simulink model "Fig32"  (R2014b)
settings: Solver=ode3  StartTime=0.0  StopTime=.005  FixedStep=2e-5  RelTol=1e-3
undefined symbols (not defined in the file or in its folder): tau
libraries: commfilt2 x2
settings Model: Creator=Dennis Silage  LastModifiedBy=Silage
settings DataIOCC: SignalLoggingSaveFormat=ModelDataLogs
settings OptimizationCC: ExpressionDepthLimit=2147483647  InitFltsAndDblsToZero=on
settings DebuggingCC: UnderspecifiedInitializationDetection=Classic  MergeDetectMultiDrivingBlocksExec=none  FcnCallInpInsideContextMsg=UseLocalSettings  StateNameClashWarn=warning  StrictBusMsg=Warning
settings GRTTargetCC: CombineOutputUpdateFcns=off  GRTInterface=on

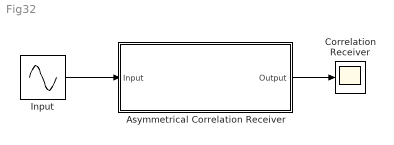
== system Fig32 ==
  "Asymmetrical Correlation Receiver " : Subsystem
  Correlation Receiver : Scope
      settings: YMin=0  YMax=30
  Input : Sin  Frequency=3141.5926  SampleTime=20e-6
  wires:
  Input/1 -> "Asymmetrical Correlation Receiver "/1(Input)
  "Asymmetrical Correlation Receiver "/1(Output) -> Correlation Receiver/1

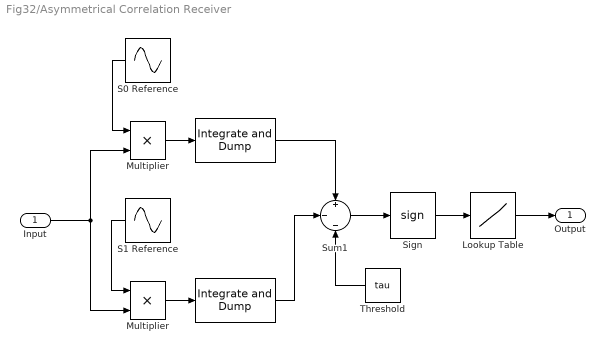
== system Fig32/Asymmetrical Correlation Receiver  ==
  Input : Inport
  " " : commfilt2/Integrate and Dump  obssamples=50  offsetsamples=0  nodump=off  roundingMode=Floor  overflowMode=off
  "   " : commfilt2/Integrate and Dump  obssamples=50  offsetsamples=0  nodump=off  roundingMode=Floor  overflowMode=off
  Lookup Table : Lookup  InputValues=[-1,0,1]  Table=[-1,-1,1]
  Multiplier : Product  RndMeth=Zero
  "Multiplier " : Product  RndMeth=Zero
  S0 Reference : Sin  Frequency=3141.59  SampleTime=20e-6  VectorParams1D=off
  S1 Reference : Sin  Frequency=3141.59  SampleTime=20e-6  VectorParams1D=off
  Sign : Signum
  Sum1 : Sum  Inputs=+|-|-
  Threshold : Constant  Value=tau
  Output : Outport
  wires:
  Multiplier/1 -> " "/1
  S0 Reference/1 -> Multiplier/1
  Input/1 -> Multiplier/2, "Multiplier "/2
  Sign/1 -> Lookup Table/1
  "Multiplier "/1 -> "   "/1
  Sum1/1 -> Sign/1
  Lookup Table/1 -> Output/1
  S1 Reference/1 -> "Multiplier "/1
  "   "/1 -> Sum1/2
  Threshold/1 -> Sum1/3
  " "/1 -> Sum1/1
